simulink model "Snake_Robot_v2_wheels_test"  (R2022b)
settings: Solver=VariableStepAuto  StartTime=0.0  StopTime=300  RelTol=1e-5  AbsTol=1e-3  EnableMultiTasking=on
values from neighbouring files (symbols this model uses):
  amplitude = 2.5    [Snake_robot_parameters.m]
  frequency = 2    [Snake_robot_parameters.m]
  phase = 1.4    [Snake_robot_parameters.m]
undefined symbols (not defined in the file or in its folder): sigbuilder_block, X, Y, Z
libraries: sm_lib x134, nesl_utility x34, simulink x5, slpidlib x5, robotalgslib x1
(part 1 of 3)
settings Model: Creator=Antoine Masson  LastModifiedBy=Antoine Masson
settings SolverCC: AutoScaleAbsTol=off  MaxZcPerStep=1
settings DataIOCC: LimitDataPoints=on  MaxDataPoints=10000
settings OptimizationCC: LifeSpan=inf
settings DebuggingCC: UnconnectedInputMsg=warning  UnconnectedOutputMsg=warning  UnconnectedLineMsg=warning  AllowSymbolicDim=off  SFUnexpectedBacktrackingDiag=warning  SFNoUnconditionalDefaultTransitionDiag=warning  SFExecutionAtInitializationDiag=none  SFMachineParentedDataDiag=warning  ArithmeticOperatorsInVariantConditions=warning
settings ModelReferenceCC: EnableRefExpFcnMdlSchedulingChecks=on
settings SFSimCC: SimUseLocalCustomCode=off  CustomCodeUndefinedFunction=UseInterfaceOnly
settings RTWCC: RTWUseLocalCustomCode=off  DLArmComputeVersion=19.05
settings CodeAppCC: StateflowObjectComments=on
settings GRTTargetCC: TargetLangStandard=C89/C90 (ANSI)
settings ConfigComp: CovMetricSettings=dw  CovSaveCumulativeToWorkspaceVar=on  CovSaveSingleToWorkspaceVar=on  CovExternalEMLEnable=off  CovSFcnEnable=off
settings SimscapeCC: SimscapeLogType=all  SimscapeLogSimulationStatistics=on  SimscapeLogDataHistory=10000

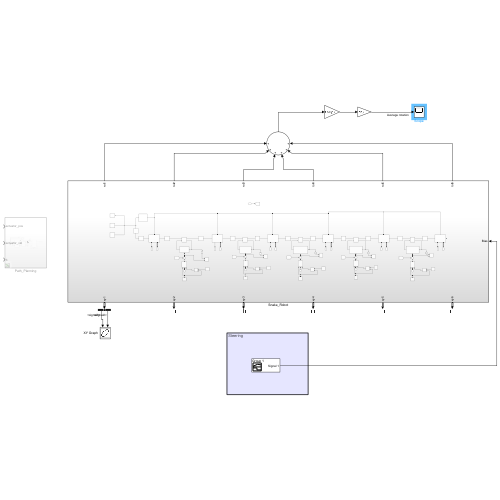
[thumbnail: Simulink's stored preview of the top-level diagram]
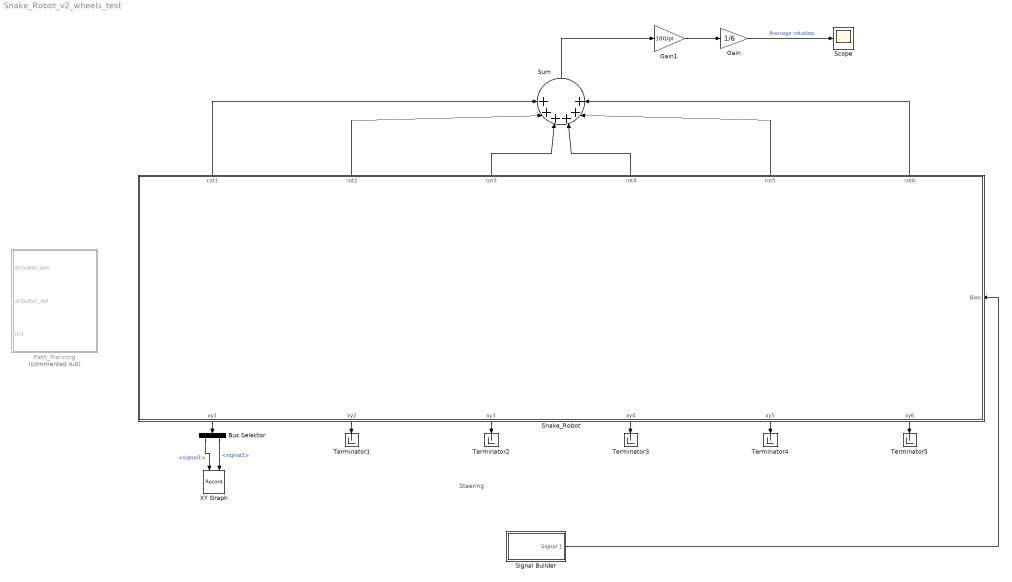
== system Snake_Robot_v2_wheels_test ==
  note: Steering
  Bus Selector : BusSelector  OutputSignals=signal1,signal2
  Gain : Gain  Gain=1/6
  Gain1 : Gain  Gain=180/pi
  Path_Planning : Subsystem  Commented=on
  Scope : Scope
  Signal Builder : Subsystem  Tag=STV Subsys  LoadFcn=sigbuilder_block('load');  StartFcn=sigbuilder_block('start');  StopFcn=sigbuilder_block('stop');  ClipboardFcn=sigbuilder_block('clipboard');  mask(Sigbuilder block){tuvar=[0:10]}
      mask help: Simulink:masks:SigbuilderBlock_MD
      mask init:
      | if ~strcmp(get_param(bdroot(gcbh),'SimulationStatus'),'stopped') tuvar = sigbuilder_block('maskInit'); end
      settings: CopyFcn=sigbuilder_block('copy');  DeleteFcn=sigbuilder_block('delete');  ModelCloseFcn=sigbuilder_block('modelClose');  PreSaveFcn=sigbuilder_block('preSave');  PauseFcn=sigbuilder_block('pause');  ContinueFcn=sigbuilder_block('continue');  NameChangeFcn=sigbuilder_block('namechange');  OpenFcn=sigbuilder_block('open',[407.4 143.4 550.8 400.2 ]);  CloseFcn=sigbuilder_block('close');
      mask Display: plot(0, 0, 100, 100,[2, 2, 32, 32, 2], [68, 8, 8, 68, 68],[32, 2], [38, 38], [32, 19, 2],[53, 60, 44], [32, 17, 17, 2],[16, 16, 31, 31]);txt = getActiveGroup(gcbh);text(2, 100, txt,'verticalAlignment', 'top');
  Snake_Robot : Subsystem
      settings: PortSchema="{\"entries\":[{\"content\":{\"sides\":[{\"content\":{\"connectorIds\":[]},\"type\":\"ConnectorPlacement.EquallySpacedRectSide\",\"uuid\":\"c8c3f42f-16ea-4b52-929c-6831ad7a0aa6\"},{\"content\":{\"connectorIds\":[\"In1\"],\"side\":\"RIGHT\"},\"type\":\"ConnectorPlacement.EquallySpacedRectSide\",\"uuid\":\"4df7dcd2-c9b7-4490-9994-4055ff239bfb\"},{\"content\":{\"connectorIds\":[\"Out7\",\"Out8\",\"Out9\",\"Out10\",\"Out11\",\"Out12\"],\"side\":\"TOP\"},\"type\":\"ConnectorPlacement.EquallySpacedRectSide\",\"uuid\":\"6c08f5c9-0650-48d0-8f84-c45eeca917d4\"},{\"content\":{\"connectorIds\":[\"Out1\",\"Out2\",\"Out3\",\"Out4\",\"Out5\",\"Out6\"],\"side\":\"BOTTOM\"},\"type\":\"ConnectorPlacement.EquallySpacedRectSide\",\"uuid\":\"57707fcd-8f3b-408f-aca2-991ac01d1cc1\"}]},\"type\":\"ConnectorPlacement.EquallySpacedConnector\",\"uuid\":\"e658f8a1-1b88-43a7-b7d0-c2a91e6742b3\"}],\"packageUris\":[\"http://schema.mathworks.com/mf0/Connector/R2020b\"],\"version\":\"1.0\"}"
  Sum : Sum  Inputs=++++++
  Terminator{1..5} (5 alike) : Terminator
  XY Graph : Record  FileSettingsInternal="{\"entries\":[{\"content\":{\"excelSettings\":{\"content\":{},\"type\":\"Streamout.ExcelSettings\"}},\"type\":\"Streamout.FileSettingStorage\",\"uuid\":\"84e75361-550c-4476-9ed0-9b3ec4275fe3\"}],\"packageUris\":[\"http://schema.mathworks.com/mf0/streamout_blocks/R2020a\"],\"version\":\"1.0\"}"  Layout=[1 1]  SignalsInternal="{\"entries\":[{\"content\":{\"signals\":[{\"content\":{\"blockPath\":[\"Snake_Robot_v2_wheels_test/XY Graph\"],\"channel\":[],\"dimensions\":[1,1],\"domain\":\"Snake_Robot_v2_wheels_test/XY Graph\",\"lineColor\":\"#a2142f\",\"plots\":[1],\"port\":1,\"sid\":[\"\"],\"signalID\":51,\"signalName\":\"<signal1>\"},\"type\":\"RecordBlkView.Signal\",\"uuid\":\"4d76fd36-35a8-4129-8bfe-1a376abbe28c\"},{\"content\":{\"blockPath\":[\"Snake_Robot_v2_wheels_test/XY Graph\"],\"channel\":[],\"dimensions\":[1,1],\"domain\":\"Snake_Robot_v2_wheels_test/XY Graph\",\"lineColor\":\"#139fff\",\"plots\":[1],\"port\":2,\"sid\":[\"\"],\"signalID\":56,\"signalName\":\"<signal2>\"},\"type\":\"RecordBlkView.Signal\",\"uuid\":\"5b063d72-9b00-41f5-95b4-b99475b325a9\"}]},\"type\":\"RecordBlkView.InputSignals\",\"uuid\":\"10acdae6-4853-4f6f-9407-9f8053fa8a6d\"}],\"packageUris\":[\"http://schema.mathworks.com/mf0/streamout_blocks/R2020a\"],\"version\":\"1.0\"}"  VisualizationBindings="{\"xyplotplugin\":{\"info\":[{\"series\":[{\"bindingParametersList\":[{\"parameter\":\"X-Axis\",\"signalID\":51,\"signalName\":\"<signal1>\"},{\"parameter\":\"Y-Axis\",\"signalID\":56,\"signalName\":\"<signal2>\"}],\"seriesID\":31576}],\"subplotID\":1}]}}"  CompatibilityTag=XY
  wires:
  Signal Builder/1(Signal 1) -> Snake_Robot/1(Bias)
  Sum/1 -> Gain1/1
  Snake_Robot/7(rot1) -> Sum/1
  Snake_Robot/8(rot2) -> Sum/2
  Snake_Robot/9(rot3) -> Sum/3
  Snake_Robot/10(rot4) -> Sum/4
  Snake_Robot/11(rot5) -> Sum/5
  Snake_Robot/12(rot6) -> Sum/6
  Snake_Robot/1(xy1) -> Bus Selector/1
  Snake_Robot/2(xy2) -> Terminator1/1
  Snake_Robot/3(xy3) -> Terminator2/1
  Snake_Robot/4(xy4) -> Terminator3/1
  Snake_Robot/5(xy5) -> Terminator4/1
  Snake_Robot/6(xy6) -> Terminator5/1
  Gain/1 -> Scope/1  "Average rotation"
  Gain1/1 -> Gain/1
  Bus Selector/1 -> XY Graph/1  "<signal1>"
  Bus Selector/2 -> XY Graph/2  "<signal2>"

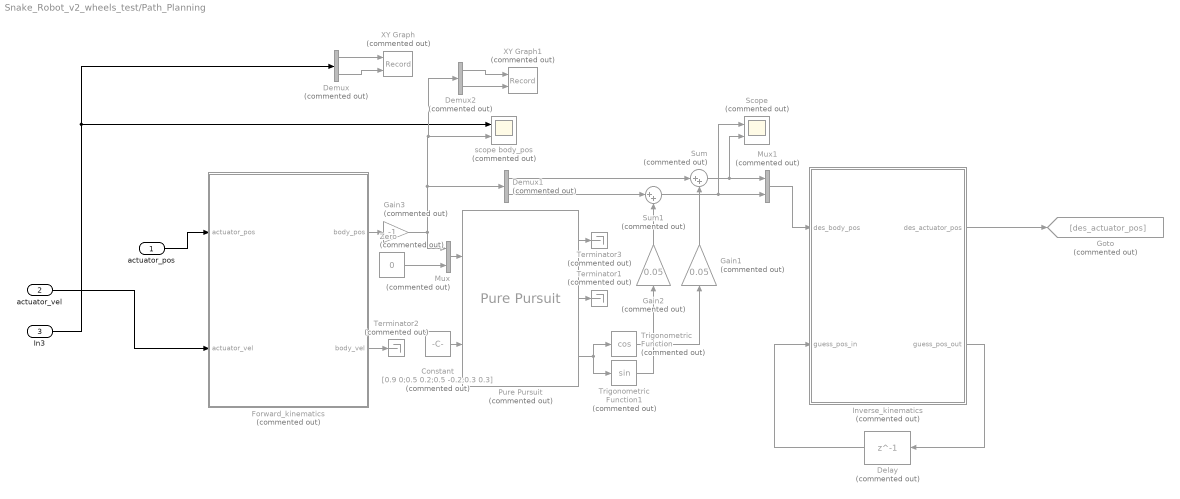
== system Snake_Robot_v2_wheels_test/Path_Planning ==
  actuator_pos : Inport
  actuator_vel : Inport  Port=2
  In3 : Inport  Port=3
  Constant : Constant  Commented=on  Value=[0.9 0;0.5 0.2;0.5 -0.2;0.3 0.3]
  Delay : Delay  Commented=on  DelayLength=1  InitialCondition=zeros(3,1)  SampleTime=0.01
  Demux : Demux  Commented=on  Outputs=2
  Demux1 : Demux  Commented=on  Outputs=2
  Demux2 : Demux  Commented=on  Outputs=2
  Forward_kinematics : MATLAB Function  Commented=on  TreatAsAtomicUnit=on
  Gain1 : Gain  Commented=on  Gain=0.05
  Gain2 : Gain  Commented=on  Gain=0.05
  Gain3 : Gain  Commented=on  Gain=-1
  Goto : Goto  Commented=on  GotoTag=des_actuator_pos
  Inverse_kinematics : MATLAB Function  Commented=on  TreatAsAtomicUnit=on
  Mux : Mux  Commented=on  Inputs=2
  Mux1 : Mux  Commented=on  Inputs=2
  Pure Pursuit : robotalgslib/Pure Pursuit  Commented=on  DesiredLinearVelocity=0.05  MaxAngularVelocity=1  LookaheadDistance=0.05  TargetDirPort=on  SimulateUsing=Code generation
      settings: LibrarySourceBlock=navlib/Control Algorithms/Pure Pursuit
  Scope : Scope  Commented=on  NumInputPorts=2
  Sum : Sum  Commented=on  Inputs=|++
  Sum1 : Sum  Commented=on  Inputs=|++
  Terminator1 : Terminator  Commented=on
  Terminator2 : Terminator  Commented=on
  Terminator3 : Terminator  Commented=on
  Trigonometric Function : Trigonometry  Commented=on  Operator=cos
  Trigonometric Function1 : Trigonometry  Commented=on
  XY Graph : Record  Commented=on  FileSettingsInternal="{\"entries\":[{\"content\":{\"excelSettings\":{\"content\":{},\"type\":\"Streamout.ExcelSettings\"}},\"type\":\"Streamout.FileSettingStorage\",\"uuid\":\"73da843e-60dd-4a33-b665-f9131d8271e1\"}],\"packageUris\":[\"http://schema.mathworks.com/mf0/streamout_blocks/R2020a\"],\"version\":\"1.0\"}"  Layout=[1 1]  SignalsInternal="{\"entries\":[{\"content\":{\"signals\":[{\"content\":{\"blockPath\":[\"Snake_Robot_v2_wheels_test/Path_Planning/XY Graph\"],\"channel\":[],\"dimensions\":[1],\"domain\":\"Snake_Robot_v2_wheels_test/Path_Planning/XY Graph\",\"lineColor\":\"#a2142f\",\"plots\":[1],\"port\":1,\"sid\":[],\"signalID\":16,\"signalName\":\"Demux:1\"},\"type\":\"RecordBlkView.Signal\",\"uuid\":\"8e68c205-c0fd-447d-ace0-da6efb5c1fbf\"},{\"content\":{\"blockPath\":[\"Snake_Robot_v2_wheels_test/Path_Planning/XY Graph\"],\"channel\":[],\"dimensions\":[1],\"domain\":\"Snake_Robot_v2_wheels_test/Path_Planning/XY Graph\",\"lineColor\":\"#139fff\",\"plots\":[1],\"port\":2,\"sid\":[],\"signalID\":19,\"signalName\":\"Demux:2\"},\"type\":\"RecordBlkView.Signal\",\"uuid\":\"8eb45edb-93bd-48a6-8f31-f79372ca3dc9\"}]},\"type\":\"RecordBlkView.InputSignals\",\"uuid\":\"d43a9e34-8350-459e-ae19-866886e7c1fb\"}],\"packageUris\":[\"http://schema.mathworks.com/mf0/streamout_blocks/R2020a\"],\"version\":\"1.0\"}"  VisualizationBindings="{\"xyplotplugin\":{\"info\":[{\"series\":[{\"bindingParametersList\":[{\"parameter\":\"X-Axis\",\"signalID\":16,\"signalName\":\"Demux:1\"},{\"parameter\":\"Y-Axis\",\"signalID\":19,\"signalName\":\"Demux:2\"}],\"seriesID\":12260}],\"subplotID\":1}]}}"  CompatibilityTag=XY
  XY Graph1 : Record  Commented=on  FileSettingsInternal="{\"entries\":[{\"content\":{\"excelSettings\":{\"content\":{},\"type\":\"Streamout.ExcelSettings\"}},\"type\":\"Streamout.FileSettingStorage\",\"uuid\":\"52cbc1bb-b168-4d3a-81e4-39640940caf6\"}],\"packageUris\":[\"http://schema.mathworks.com/mf0/streamout_blocks/R2020a\"],\"version\":\"1.0\"}"  Layout=[1 1]  SignalsInternal="{\"entries\":[{\"content\":{\"signals\":[{\"content\":{\"blockPath\":[\"Snake_Robot_v2_wheels_test/Path_Planning/XY Graph1\"],\"channel\":[],\"dimensions\":[1,1],\"domain\":\"Snake_Robot_v2_wheels_test/Path_Planning/XY Graph1\",\"lineColor\":\"#a2142f\",\"plots\":[1],\"port\":1,\"sid\":[],\"signalID\":8,\"signalName\":\"Demux2:1\"},\"type\":\"RecordBlkView.Signal\",\"uuid\":\"6807b1ac-bdd6-4ace-a695-6e3cb940d5f2\"},{\"content\":{\"blockPath\":[\"Snake_Robot_v2_wheels_test/Path_Planning/XY Graph1\"],\"channel\":[],\"dimensions\":[1,1],\"domain\":\"Snake_Robot_v2_wheels_test/Path_Planning/XY Graph1\",\"lineColor\":\"#139fff\",\"plots\":[1],\"port\":2,\"sid\":[],\"signalID\":11,\"signalName\":\"Demux2:2\"},\"type\":\"RecordBlkView.Signal\",\"uuid\":\"ed18573f-74af-480a-a61e-83f3faac892a\"}]},\"type\":\"RecordBlkView.InputSignals\",\"uuid\":\"ad915e20-bbb1-4588-94b6-02e62a7d6124\"}],\"packageUris\":[\"http://schema.mathworks.com/mf0/streamout_blocks/R2020a\"],\"version\":\"1.0\"}"  VisualizationBindings="{\"xyplotplugin\":{\"info\":[{\"series\":[{\"bindingParametersList\":[{\"parameter\":\"X-Axis\",\"signalID\":8,\"signalName\":\"Demux2:1\"},{\"parameter\":\"Y-Axis\",\"signalID\":11,\"signalName\":\"Demux2:2\"}],\"seriesID\":53918}],\"subplotID\":1}]}}"  CompatibilityTag=XY
  Zero : Constant  Commented=on  Value=0  OutDataTypeStr=Inherit: Inherit via back propagation
  scope body_pos : Scope  Commented=on  NumInputPorts=2
  wires:
  Forward_kinematics/1(body_pos) -> Gain3/1
  Trigonometric Function/1 -> Gain1/1
  Demux1/2 -> Sum1/1
  Sum/1 -> Scope/2, Mux1/1
  Inverse_kinematics/1(des_actuator_pos) -> Goto/1
  Constant/1 -> Pure Pursuit/2
  Pure Pursuit/3 -> Trigonometric Function/1, Trigonometric Function1/1
  Mux/1 -> Pure Pursuit/1
  In3/1 -> Demux/1, scope body_pos/1
  Mux1/1 -> Inverse_kinematics/1(des_body_pos)
  Forward_kinematics/2(body_vel) -> Terminator2/1
  Demux2/1 -> XY Graph1/1
  Sum1/1 -> Scope/1, Mux1/2
  Gain2/1 -> Sum1/2
  Gain1/1 -> Sum/2
  Trigonometric Function1/1 -> Gain2/1
  Delay/1 -> Inverse_kinematics/2(guess_pos_in)
  actuator_vel/1 -> Forward_kinematics/2(actuator_vel)
  Inverse_kinematics/2(guess_pos_out) -> Delay/1
  Gain3/1 -> Mux/1, Demux2/1, scope body_pos/2, Demux1/1
  Demux1/1 -> Sum/1
  Zero/1 -> Mux/2
  Pure Pursuit/2 -> Terminator1/1
  Demux2/2 -> XY Graph1/2
  Pure Pursuit/1 -> Terminator3/1
  Demux/1 -> XY Graph/1
  Demux/2 -> XY Graph/2
  actuator_pos/1 -> Forward_kinematics/1(actuator_pos)

== system Snake_Robot_v2_wheels_test/Signal Builder ==
  Demux : Demux  Tag=STV Demux  Outputs=1
      settings: DisplayOption=none
  FromWs : FromWorkspace  Tag=STV FromWs  VariableName=tuvar
      SigBuilderData=|
      | common.afterFinalStr = 'Extrapolate'
      | common.sampleTime = 0
      | dataSet.timeRange = [0 60]
      | dataSet.name = 'Group 1'
      | sbobj.Groups.Name = 'Group 1'
      | sbobj.Groups.Signals.Name = 'Signal 1'
      | sbobj.Groups.Signals.XData = [0 15 19 23 35 40 45 60]
      | sbobj.Groups.Signals.YData = [0 0 -0.3 0 0 0.3 0 0]
      | sbobj.Groups.TimeRange = [0 60]
  Signal 1 : Outport  Tag=STV Outport
  wires:
  Demux/1 -> Signal 1/1
  FromWs/1 -> Demux/1

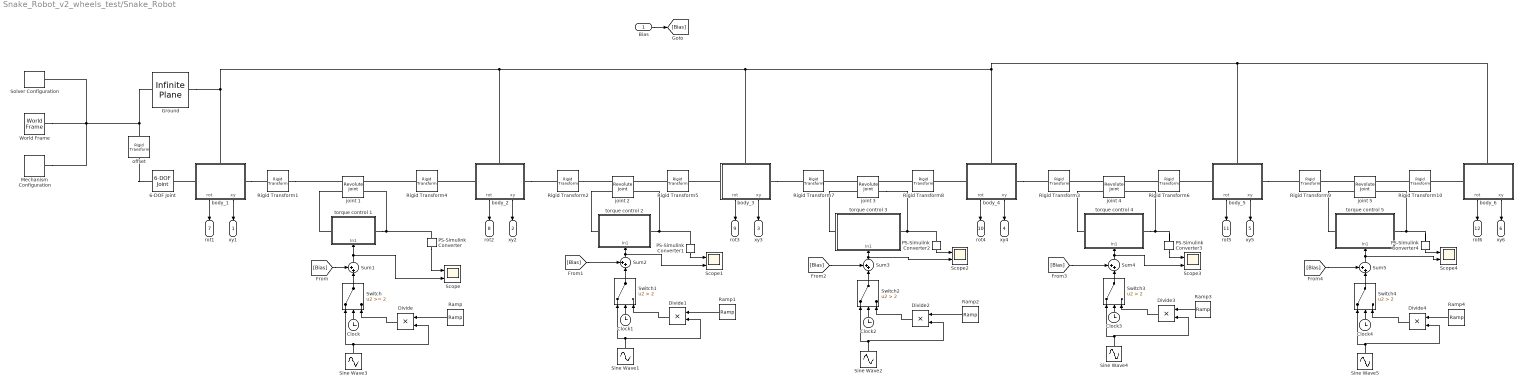
== system Snake_Robot_v2_wheels_test/Snake_Robot ==
  Bias : Inport
  6-DOF Joint : sm_lib/Joints/6-DOF Joint  JointMode=Normal  SenseConstraintForce=off  SenseConstraintForceX=off  SenseConstraintForceY=off  SenseConstraintForceZ=off  SenseConstraintTorque=off  SenseConstraintTorqueX=off  SenseConstraintTorqueY=off  SenseConstraintTorqueZ=off  SenseTotalForce=off  SenseTotalForceX=off  SenseTotalForceY=off  SenseTotalForceZ=off  SenseTotalTorque=off  SenseTotalTorqueX=off  SenseTotalTorqueY=off  SenseTotalTorqueZ=off  CompositeWrenchDir=FollowerOnBase  CompositeWrenchFrame=BaseFrame  PxEquilibriumPosition=0  PxEquilibriumPositionUnits=m  PxSpringStiffness=0  PxSpringStiffnessUnits=N/m  PxDampingCoefficient=0  PxDampingCoefficientUnits=N/(m/s)  PxTorqueActuationMode=NoTorque  PxMotionActuationMode=ComputedMotion  PxSensePosition=off  PxSenseVelocity=off  PxSenseAcceleration=off  PxSenseTorqueForce=off  PxSenseLowerLimitTorqueForce=off  PxSenseUpperLimitTorqueForce=off  PxLowerLimitSpecify=off  PxLowerLimitBound=-1  PxLowerLimitBoundUnits=m  PxLowerLimitStiffness=1e6  PxLowerLimitStiffnessUnits=N/m  PxLowerLimitDamping=1e3  PxLowerLimitDampingUnits=N/(m/s)  PxLowerLimitTransitionRegionWidth=1e-4  PxLowerLimitTransitionRegionWidthUnits=m  PxUpperLimitSpecify=off  PxUpperLimitBound=1  PxUpperLimitBoundUnits=m  PxUpperLimitStiffness=1e6  PxUpperLimitStiffnessUnits=N/m  PxUpperLimitDamping=1e3  PxUpperLimitDampingUnits=N/(m/s)  PxUpperLimitTransitionRegionWidth=1e-4  PxUpperLimitTransitionRegionWidthUnits=m  PxPositionTargetSpecify=off  PxPositionTargetPriority=High  PxPositionTargetValue=0  PxPositionTargetValueUnits=m  PxVelocityTargetSpecify=off  PxVelocityTargetPriority=High  PxVelocityTargetValue=0  PxVelocityTargetValueUnits=m/s  PyEquilibriumPosition=0  PyEquilibriumPositionUnits=m  PySpringStiffness=0  PySpringStiffnessUnits=N/m  PyDampingCoefficient=0  PyDampingCoefficientUnits=N/(m/s)  PyTorqueActuationMode=NoTorque  PyMotionActuationMode=ComputedMotion  PySensePosition=off  PySenseVelocity=off  PySenseAcceleration=off  PySenseTorqueForce=off  PySenseLowerLimitTorqueForce=off  PySenseUpperLimitTorqueForce=off  PyLowerLimitSpecify=off  PyLowerLimitBound=-1  PyLowerLimitBoundUnits=m  PyLowerLimitStiffness=1e6  PyLowerLimitStiffnessUnits=N/m  PyLowerLimitDamping=1e3  PyLowerLimitDampingUnits=N/(m/s)  PyLowerLimitTransitionRegionWidth=1e-4  PyLowerLimitTransitionRegionWidthUnits=m  PyUpperLimitSpecify=off  PyUpperLimitBound=1  PyUpperLimitBoundUnits=m  PyUpperLimitStiffness=1e6  PyUpperLimitStiffnessUnits=N/m  PyUpperLimitDamping=1e3  PyUpperLimitDampingUnits=N/(m/s)  PyUpperLimitTransitionRegionWidth=1e-4  PyUpperLimitTransitionRegionWidthUnits=m  PyPositionTargetSpecify=off  PyPositionTargetPriority=High  PyPositionTargetValue=0  PyPositionTargetValueUnits=m  PyVelocityTargetSpecify=off  PyVelocityTargetPriority=High  PyVelocityTargetValue=0  PyVelocityTargetValueUnits=m/s  PzEquilibriumPosition=0  PzEquilibriumPositionUnits=m  PzSpringStiffness=0  PzSpringStiffnessUnits=N/m  PzDampingCoefficient=0  PzDampingCoefficientUnits=N/(m/s)  PzTorqueActuationMode=NoTorque  PzMotionActuationMode=ComputedMotion  PzSensePosition=off  PzSenseVelocity=off  PzSenseAcceleration=off  PzSenseTorqueForce=off  PzSenseLowerLimitTorqueForce=off  PzSenseUpperLimitTorqueForce=off  PzLowerLimitSpecify=off  PzLowerLimitBound=-1  PzLowerLimitBoundUnits=m  PzLowerLimitStiffness=1e6  PzLowerLimitStiffnessUnits=N/m  PzLowerLimitDamping=1e3  PzLowerLimitDampingUnits=N/(m/s)  PzLowerLimitTransitionRegionWidth=1e-4  PzLowerLimitTransitionRegionWidthUnits=m  PzUpperLimitSpecify=off  PzUpperLimitBound=1  PzUpperLimitBoundUnits=m  PzUpperLimitStiffness=1e6  PzUpperLimitStiffnessUnits=N/m  PzUpperLimitDamping=1e3  PzUpperLimitDampingUnits=N/(m/s)  PzUpperLimitTransitionRegionWidth=1e-4  PzUpperLimitTransitionRegionWidthUnits=m  PzPositionTargetSpecify=off  PzPositionTargetPriority=High  PzPositionTargetValue=0  PzPositionTargetValueUnits=m  PzVelocityTargetSpecify=off  PzVelocityTargetPriority=High  PzVelocityTargetValue=0  PzVelocityTargetValueUnits=m/s  SphEqPosRotationMethod=None  SphEqPosRotationAngleUnits=deg  SphEqPosRotationStandardAxis=+Z  SphEqPosRotationAngle=0.0  SphEqPosRotationArbitraryAxis=[0 0 1]  SphEqPosFollAlignAxisA=+X  SphEqPosBaseAlignAxisA=+Y  SphEqPosFollAlignAxisB=+Y  SphEqPosBaseAlignAxisB=+Z  SphEqPosRotationSequenceAxes=FollowerAxes  SphEqPosRotationSequence=XYX  SphEqPosRotationSequenceAngles=[0 0 0]  SphEqPosRotationSequenceAnglesUnits=deg  SphEqPosRotationMatrix=[1 0 0; 0 1 0; 0 0 1]  SphEqPosQuaternion=[1 0 0 0]  SphSpringStiffness=0  SphSpringStiffnessUnits=N*m/deg  SphDampingCoefficient=0  SphDampingCoefficientUnits=N*m/(deg/s)  SphActuateTorqueX=off  SphActuateTorqueY=off  SphActuateTorqueZ=off  SphActuateTorque=off  SphTorqueActuationMode=NoTorque  SphMotionActuationMode=ComputedMotion  SphActuationFrame=BaseFrame  SphSensePosition=off  SphSenseVelocityX=off  SphSenseVelocityY=off  SphSenseVelocityZ=off  SphSenseVelocity=off  SphSenseAccelerationX=off  SphSenseAccelerationY=off  SphSenseAccelerationZ=off  SphSenseAcceleration=off  SphSenseTorqueX=off  SphSenseTorqueY=off  SphSenseTorqueZ=off  SphSenseTorqueForce=off  SphSenseLowerLimitTorqueMag=off  SphSenseUpperLimitTorqueMag=off  SphSensingFrame=BaseFrame  SphLowerLimitSpecify=off  SphLowerLimitBound=15  SphLowerLimitBoundUnits=deg  SphLowerLimitStiffness=1e4  SphLowerLimitStiffnessUnits=N*m/deg  SphLowerLimitDamping=10  SphLowerLimitDampingUnits=N*m/(deg/s)  SphLowerLimitTransitionRegionWidth=0.1  SphLowerLimitTransitionRegionWidthUnits=deg  SphUpperLimitSpecify=off  SphUpperLimitBound=45  SphUpperLimitBoundUnits=deg  SphUpperLimitStiffness=1e4  SphUpperLimitStiffnessUnits=N*m/deg  SphUpperLimitDamping=10  SphUpperLimitDampingUnits=N*m/(deg/s)  SphUpperLimitTransitionRegionWidth=0.1  SphUpperLimitTransitionRegionWidthUnits=deg  SphPositionTargetRotationMethod=None  SphPositionTargetRotationAngleUnits=deg  SphPositionTargetRotationStandardAxis=+Z  SphPositionTargetRotationAngle=0.0  SphPositionTargetRotationArbitraryAxis=[0 0 1]  SphPositionTargetFollAlignAxisA=+X  SphPositionTargetBaseAlignAxisA=+Y  SphPositionTargetFollAlignAxisB=+Y  SphPositionTargetBaseAlignAxisB=+Z  SphPositionTargetRotationSequenceAxes=FollowerAxes  SphPositionTargetRotationSequence=XYX  SphPositionTargetRotationSequenceAngles=[0 0 0]  SphPositionTargetRotationSequenceAnglesUnits=deg  SphPositionTargetRotationMatrix=[1 0 0; 0 1 0; 0 0 1]  SphPositionTargetQuaternion=[1 0 0 0]  SphPositionTargetSpecify=off  SphPositionTargetPriority=High  SphVelocityTargetValue=[0 0 0]  SphVelocityTargetValueUnits=deg/s  SphVelocityTargetSpecify=off  SphVelocityTargetPriority=High  SphVelocityTargetInFollowerFrame=on
  Clock{,1..4} (5 alike) : Clock
  Divide{,1..4} (5 alike) : Product  Inputs=**
  Ground : sm_lib/Curves and Surfaces/Infinite Plane  GraphicType=Rectangle  GraphicPlaneWidth=20  GraphicPlaneWidthUnits=m  GraphicPlaneHeight=20  GraphicPlaneHeightUnits=m  GraphicVisPropType=SimpleVisualProperties  GraphicDiffuseColor=[1 1 1]  GraphicOpacity=1  GraphicSpecularColor=[0.5 0.5 0.5 1.0]  GraphicAmbientColor=[0.15 0.15 0.15 1.0]  GraphicEmissiveColor=[0.0 0.0 0.0 1.0]  GraphicShininess=75
  Mechanism Configuration : sm_lib/Utilities/Mechanism Configuration  UniformGravity=Constant  GravityVector=[0 0 -9.80665]  GravityUnits=m/s^2  LinearizationDelta=0.001  JointModeTransitionNonlinearIterations=2
  PS-Simulink Converter{,1..4} (5 alike) : nesl_utility/PS-Simulink Converter  PhysicalDomain=network_engine_domain  SubClassName=ps_output  LeftPortType=input  RightPortType=output  PseudoPeriodic=off  Frequencies=[]  VectorFormat=inherit  Unit=inherit  AffineConversion=off
  Ramp{,1..4} (5 alike) : simulink/Sources/Ramp  slope=0.5  start=0  InitialOutput=0
  Rigid Transform{1..10} (10 alike) : sm_lib/Frames and Transforms/Rigid Transform  TranslationMethod=Cartesian  TranslationStandardOffset=0  TranslationLengthUnit=m  TranslationStandardAxis=+Z  TranslationCartesianOffset=[0.05 0 0]  TranslationROffset=0  TranslationROffsetUnits=m  TranslationZOffset=0  TranslationZOffsetUnits=m  TranslationThetaOffset=0  TranslationThetaOffsetUnits=deg  RotationMethod=None  RotationAngleUnits=deg  RotationStandardAxis=+Z  RotationAngle=0.0  RotationArbitraryAxis=[0 0 1]  FollAlignAxisA=+X  BaseAlignAxisA=+Y  FollAlignAxisB=+Y  BaseAlignAxisB=+Z  RotationSequenceAxes=FollowerAxes  RotationSequence=XYX  RotationSequenceAngles=[0 0 0]  RotationSequenceAnglesUnits=deg  RotationMatrix=[1 0 0; 0 1 0; 0 0 1]  Quaternion=[1 0 0 0]
  Scope{,1..4} (5 alike) : Scope  NumInputPorts=2
  Sine Wave1 : Sin  Amplitude=amplitude  Frequency=frequency  Phase=1*phase  SampleTime=0.01
  Sine Wave2 : Sin  Amplitude=amplitude  Frequency=frequency  Phase=2*phase  SampleTime=0.01
  Sine Wave3 : Sin  Amplitude=amplitude  Frequency=frequency  Phase=0*phase  SampleTime=0.01
  Sine Wave4 : Sin  Amplitude=amplitude  Frequency=frequency  Phase=3*phase  SampleTime=0.01
  Sine Wave5 : Sin  Amplitude=amplitude  Frequency=frequency  Phase=4*phase  SampleTime=0.01
  Solver Configuration : nesl_utility/Solver Configuration  PhysicalDomain=network_engine_domain  SubClassName=solver  LeftPortType=input  RightPortType=generic  Tones=[]  Harmonics=[]  SimulateNoise=off  Profile=off  UseLocalSampling=off  EnableSwitchedLinearOptims=on  FrequencyDomain=off  UseCCode=off  RelTol=0.001  AbsTol=1e-06  MinStep=1e-09  ToWorkspace=off  RevertToSquareIcSolve=off  NumHomotopyIterations=100  PhasorMode=off  PhasorModeNumHarmonics=1  ConsistencySolver=NEWTON_XTOL_AFTER_FTOL  IndexReductionMethod=DerivativeReplacement  DoDC=off  ResidualTolerance=1e-09  ConsistencyTolSource=GLOBAL  ConsistencyAbsTol=0.001  ConsistencyRelTol=0.001  ConsistencyTolFactor=0.001  UseLocalSolver=off  LocalSolverChoice=NE_BACKWARD_EULER_ADVANCER  ResolveIndetEquations=on  FunctionEvalNumThread=1  LocalSolverSampleTime=0.001  DoFixedCost=off  MaxNonlinIter=3  MaxModeIter=2  ComputeImpulses=off  ImpulseIterations=2  LinearAlgebra=Sparse  LinearAlgebraNumThread=0  EquationFormulation=NE_TIME_EF  DelaysMemoryBudget=1024  AutomaticFiltering=on  FilteringTimeConstant=0.001  PartitionStorageMethod=AS_NEEDED  PartitionMemoryBudget=1024  PartitionMethod=FAST
  Sum{1..5} (5 alike) : Sum  Inputs=++|
  Switch : Switch  Threshold=2  SaturateOnIntegerOverflow=off  InputSameDT=off
  Switch{1..4} (4 alike) : Switch  Criteria=u2 > Threshold  Threshold=2  SaturateOnIntegerOverflow=off  InputSameDT=off
  World Frame : sm_lib/Frames and Transforms/World Frame
  body_1 : Subsystem
      settings: PortSchema="{\"entries\":[{\"content\":{\"sides\":[{\"content\":{\"connectorIds\":[\"LConn1\"]},\"type\":\"ConnectorPlacement.EquallySpacedRectSide\",\"uuid\":\"751caf70-fea4-4832-96d1-cfb89594f882\"},{\"content\":{\"connectorIds\":[\"RConn1\"],\"side\":\"RIGHT\"},\"type\":\"ConnectorPlacement.EquallySpacedRectSide\",\"uuid\":\"f4256cb0-7155-4962-9e91-24184222dcac\"},{\"content\":{\"connectorIds\":[\"LConn2\"],\"side\":\"TOP\"},\"type\":\"ConnectorPlacement.EquallySpacedRectSide\",\"uuid\":\"795803ba-ad55-452c-8522-189aeb3dc475\"},{\"content\":{\"connectorIds\":[\"Out1\",\"Out2\"],\"side\":\"BOTTOM\"},\"type\":\"ConnectorPlacement.EquallySpacedRectSide\",\"uuid\":\"40385723-46d7-44c7-bad8-75426342e5d4\"}]},\"type\":\"ConnectorPlacement.EquallySpacedConnector\",\"uuid\":\"3814bf41-4d16-483c-99d1-47665b43720b\"}],\"packageUris\":[\"http://schema.mathworks.com/mf0/Connector/R2020b\"],\"version\":\"1.0\"}"
  body_2 : Subsystem
      settings: PortSchema="{\"entries\":[{\"content\":{\"sides\":[{\"content\":{\"connectorIds\":[\"LConn1\"]},\"type\":\"ConnectorPlacement.EquallySpacedRectSide\",\"uuid\":\"751caf70-fea4-4832-96d1-cfb89594f882\"},{\"content\":{\"connectorIds\":[\"RConn1\"],\"side\":\"RIGHT\"},\"type\":\"ConnectorPlacement.EquallySpacedRectSide\",\"uuid\":\"f4256cb0-7155-4962-9e91-24184222dcac\"},{\"content\":{\"connectorIds\":[\"LConn2\"],\"side\":\"TOP\"},\"type\":\"ConnectorPlacement.EquallySpacedRectSide\",\"uuid\":\"795803ba-ad55-452c-8522-189aeb3dc475\"},{\"content\":{\"connectorIds\":[\"Out1\",\"Out2\"],\"side\":\"BOTTOM\"},\"type\":\"ConnectorPlacement.EquallySpacedRectSide\",\"uuid\":\"40385723-46d7-44c7-bad8-75426342e5d4\"}]},\"type\":\"ConnectorPlacement.EquallySpacedConnector\",\"uuid\":\"3814bf41-4d16-483c-99d1-47665b43720b\"}],\"packageUris\":[\"http://schema.mathworks.com/mf0/Connector/R2020b\"],\"version\":\"1.0\"}"
  body_3 : Subsystem
      settings: PortSchema="{\"entries\":[{\"content\":{\"sides\":[{\"content\":{\"connectorIds\":[\"LConn1\"]},\"type\":\"ConnectorPlacement.EquallySpacedRectSide\",\"uuid\":\"751caf70-fea4-4832-96d1-cfb89594f882\"},{\"content\":{\"connectorIds\":[\"RConn1\"],\"side\":\"RIGHT\"},\"type\":\"ConnectorPlacement.EquallySpacedRectSide\",\"uuid\":\"f4256cb0-7155-4962-9e91-24184222dcac\"},{\"content\":{\"connectorIds\":[\"LConn2\"],\"side\":\"TOP\"},\"type\":\"ConnectorPlacement.EquallySpacedRectSide\",\"uuid\":\"795803ba-ad55-452c-8522-189aeb3dc475\"},{\"content\":{\"connectorIds\":[\"Out1\",\"Out2\"],\"side\":\"BOTTOM\"},\"type\":\"ConnectorPlacement.EquallySpacedRectSide\",\"uuid\":\"40385723-46d7-44c7-bad8-75426342e5d4\"}]},\"type\":\"ConnectorPlacement.EquallySpacedConnector\",\"uuid\":\"3814bf41-4d16-483c-99d1-47665b43720b\"}],\"packageUris\":[\"http://schema.mathworks.com/mf0/Connector/R2020b\"],\"version\":\"1.0\"}"
  body_4 : Subsystem
      settings: PortSchema="{\"entries\":[{\"content\":{\"sides\":[{\"content\":{\"connectorIds\":[\"LConn1\"]},\"type\":\"ConnectorPlacement.EquallySpacedRectSide\",\"uuid\":\"751caf70-fea4-4832-96d1-cfb89594f882\"},{\"content\":{\"connectorIds\":[\"RConn1\"],\"side\":\"RIGHT\"},\"type\":\"ConnectorPlacement.EquallySpacedRectSide\",\"uuid\":\"f4256cb0-7155-4962-9e91-24184222dcac\"},{\"content\":{\"connectorIds\":[\"LConn2\"],\"side\":\"TOP\"},\"type\":\"ConnectorPlacement.EquallySpacedRectSide\",\"uuid\":\"795803ba-ad55-452c-8522-189aeb3dc475\"},{\"content\":{\"connectorIds\":[\"Out1\",\"Out2\"],\"side\":\"BOTTOM\"},\"type\":\"ConnectorPlacement.EquallySpacedRectSide\",\"uuid\":\"40385723-46d7-44c7-bad8-75426342e5d4\"}]},\"type\":\"ConnectorPlacement.EquallySpacedConnector\",\"uuid\":\"3814bf41-4d16-483c-99d1-47665b43720b\"}],\"packageUris\":[\"http://schema.mathworks.com/mf0/Connector/R2020b\"],\"version\":\"1.0\"}"
  body_5 : Subsystem
      settings: PortSchema="{\"entries\":[{\"content\":{\"sides\":[{\"content\":{\"connectorIds\":[\"LConn1\"]},\"type\":\"ConnectorPlacement.EquallySpacedRectSide\",\"uuid\":\"751caf70-fea4-4832-96d1-cfb89594f882\"},{\"content\":{\"connectorIds\":[\"RConn1\"],\"side\":\"RIGHT\"},\"type\":\"ConnectorPlacement.EquallySpacedRectSide\",\"uuid\":\"f4256cb0-7155-4962-9e91-24184222dcac\"},{\"content\":{\"connectorIds\":[\"LConn2\"],\"side\":\"TOP\"},\"type\":\"ConnectorPlacement.EquallySpacedRectSide\",\"uuid\":\"795803ba-ad55-452c-8522-189aeb3dc475\"},{\"content\":{\"connectorIds\":[\"Out1\",\"Out2\"],\"side\":\"BOTTOM\"},\"type\":\"ConnectorPlacement.EquallySpacedRectSide\",\"uuid\":\"40385723-46d7-44c7-bad8-75426342e5d4\"}]},\"type\":\"ConnectorPlacement.EquallySpacedConnector\",\"uuid\":\"3814bf41-4d16-483c-99d1-47665b43720b\"}],\"packageUris\":[\"http://schema.mathworks.com/mf0/Connector/R2020b\"],\"version\":\"1.0\"}"
  body_6 : Subsystem
      settings: PortSchema="{\"entries\":[{\"content\":{\"sides\":[{\"content\":{\"connectorIds\":[\"LConn1\"]},\"type\":\"ConnectorPlacement.EquallySpacedRectSide\",\"uuid\":\"751caf70-fea4-4832-96d1-cfb89594f882\"},{\"content\":{\"connectorIds\":[\"RConn1\"],\"side\":\"RIGHT\"},\"type\":\"ConnectorPlacement.EquallySpacedRectSide\",\"uuid\":\"f4256cb0-7155-4962-9e91-24184222dcac\"},{\"content\":{\"connectorIds\":[\"LConn2\"],\"side\":\"TOP\"},\"type\":\"ConnectorPlacement.EquallySpacedRectSide\",\"uuid\":\"795803ba-ad55-452c-8522-189aeb3dc475\"},{\"content\":{\"connectorIds\":[\"Out1\",\"Out2\"],\"side\":\"BOTTOM\"},\"type\":\"ConnectorPlacement.EquallySpacedRectSide\",\"uuid\":\"40385723-46d7-44c7-bad8-75426342e5d4\"}]},\"type\":\"ConnectorPlacement.EquallySpacedConnector\",\"uuid\":\"3814bf41-4d16-483c-99d1-47665b43720b\"}],\"packageUris\":[\"http://schema.mathworks.com/mf0/Connector/R2020b\"],\"version\":\"1.0\"}"
  joint {1..5} (5 alike) : sm_lib/Joints/Revolute Joint  JointMode=Normal  SenseConstraintForce=off  SenseConstraintForceX=off  SenseConstraintForceY=off  SenseConstraintForceZ=off  SenseConstraintTorque=off  SenseConstraintTorqueX=off  SenseConstraintTorqueY=off  SenseConstraintTorqueZ=off  SenseTotalForce=off  SenseTotalForceX=off  SenseTotalForceY=off  SenseTotalForceZ=off  SenseTotalTorque=off  SenseTotalTorqueX=off  SenseTotalTorqueY=off  SenseTotalTorqueZ=off  CompositeWrenchDir=FollowerOnBase  CompositeWrenchFrame=BaseFrame  EquilibriumPosition=0  EquilibriumPositionUnits=deg  SpringStiffness=internal_stiffness  SpringStiffnessUnits=N*m/deg  DampingCoefficient=0  DampingCoefficientUnits=N*m/(deg/s)  TorqueActuationMode=InputTorque  MotionActuationMode=ComputedMotion  SensePosition=on  SenseVelocity=off  SenseAcceleration=off  SenseTorqueForce=off  SenseLowerLimitTorqueForce=off  SenseUpperLimitTorqueForce=off  LowerLimitSpecify=on  LowerLimitBound=-90  LowerLimitBoundUnits=deg  LowerLimitStiffness=spring_stiffness  LowerLimitStiffnessUnits=N*m/deg  LowerLimitDamping=joint_damp  LowerLimitDampingUnits=N*m/(deg/s)  LowerLimitTransitionRegionWidth=0.1  LowerLimitTransitionRegionWidthUnits=deg  UpperLimitSpecify=on  UpperLimitBound=90  UpperLimitBoundUnits=deg  UpperLimitStiffness=spring_stiffness  UpperLimitStiffnessUnits=N*m/deg  UpperLimitDamping=joint_damp  UpperLimitDampingUnits=N*m/(deg/s)  UpperLimitTransitionRegionWidth=0.1  UpperLimitTransitionRegionWidthUnits=deg  PositionTargetSpecify=off  PositionTargetPriority=High  PositionTargetValue=0  PositionTargetValueUnits=deg  VelocityTargetSpecify=off  VelocityTargetPriority=High  VelocityTargetValue=0  VelocityTargetValueUnits=deg/s
  offset : sm_lib/Frames and Transforms/Rigid Transform  TranslationMethod=Cartesian  TranslationStandardOffset=0  TranslationLengthUnit=m  TranslationStandardAxis=+Z  TranslationCartesianOffset=[0 0 0.06]  TranslationROffset=0  TranslationROffsetUnits=m  TranslationZOffset=0  TranslationZOffsetUnits=m  TranslationThetaOffset=0  TranslationThetaOffsetUnits=deg  RotationMethod=None  RotationAngleUnits=deg  RotationStandardAxis=+Z  RotationAngle=0.0  RotationArbitraryAxis=[0 0 1]  FollAlignAxisA=+X  BaseAlignAxisA=+Y  FollAlignAxisB=+Y  BaseAlignAxisB=+Z  RotationSequenceAxes=FollowerAxes  RotationSequence=XYX  RotationSequenceAngles=[0 0 0]  RotationSequenceAnglesUnits=deg  RotationMatrix=[1 0 0; 0 1 0; 0 0 1]  Quaternion=[1 0 0 0]
  torque control 1 : Subsystem
      settings: PortSchema="{\"entries\":[{\"content\":{\"sides\":[{\"content\":{\"connectorIds\":[\"LConn1\"]},\"type\":\"ConnectorPlacement.EquallySpacedRectSide\",\"uuid\":\"a098fbb4-d319-4217-913e-12f869fe3f7f\"},{\"content\":{\"connectorIds\":[\"RConn1\"],\"side\":\"RIGHT\"},\"type\":\"ConnectorPlacement.EquallySpacedRectSide\",\"uuid\":\"0b47f4a1-f0fa-49d7-9b0e-df1cd63c93cc\"},{\"content\":{\"connectorIds\":[],\"side\":\"TOP\"},\"type\":\"ConnectorPlacement.EquallySpacedRectSide\",\"uuid\":\"12733803-042e-49c1-bd12-ad77a161d0eb\"},{\"content\":{\"connectorIds\":[\"In1\"],\"side\":\"BOTTOM\"},\"type\":\"ConnectorPlacement.EquallySpacedRectSide\",\"uuid\":\"dd4379fb-4796-4e85-9b1d-ab5e12fdce52\"}]},\"type\":\"ConnectorPlacement.EquallySpacedConnector\",\"uuid\":\"2c004d5d-bdbd-4eb1-9300-9454cbe520aa\"}],\"packageUris\":[\"http://schema.mathworks.com/mf0/Connector/R2020b\"],\"version\":\"1.0\"}"
  torque control 2 : Subsystem
      settings: PortSchema="{\"entries\":[{\"content\":{\"sides\":[{\"content\":{\"connectorIds\":[\"LConn1\"]},\"type\":\"ConnectorPlacement.EquallySpacedRectSide\",\"uuid\":\"b601c68f-6f7e-4b60-bd4c-7c9a60dfa343\"},{\"content\":{\"connectorIds\":[\"RConn1\"],\"side\":\"RIGHT\"},\"type\":\"ConnectorPlacement.EquallySpacedRectSide\",\"uuid\":\"26f160aa-f34c-4483-ba01-5c959bffdc56\"},{\"content\":{\"connectorIds\":[],\"side\":\"TOP\"},\"type\":\"ConnectorPlacement.EquallySpacedRectSide\",\"uuid\":\"5bc877b6-64cf-4559-a179-0d622b0df1ec\"},{\"content\":{\"connectorIds\":[\"In1\"],\"side\":\"BOTTOM\"},\"type\":\"ConnectorPlacement.EquallySpacedRectSide\",\"uuid\":\"faa2df67-1e79-4353-a2fd-6cb2d7599dbb\"}]},\"type\":\"ConnectorPlacement.EquallySpacedConnector\",\"uuid\":\"4a9b8871-07f6-45c3-a06e-bcb1a798cb73\"}],\"packageUris\":[\"http://schema.mathworks.com/mf0/Connector/R2020b\"],\"version\":\"1.0\"}"
  torque control 3 : Subsystem
      settings: PortSchema="{\"entries\":[{\"content\":{\"sides\":[{\"content\":{\"connectorIds\":[\"LConn1\"]},\"type\":\"ConnectorPlacement.EquallySpacedRectSide\",\"uuid\":\"a098fbb4-d319-4217-913e-12f869fe3f7f\"},{\"content\":{\"connectorIds\":[\"RConn1\"],\"side\":\"RIGHT\"},\"type\":\"ConnectorPlacement.EquallySpacedRectSide\",\"uuid\":\"0b47f4a1-f0fa-49d7-9b0e-df1cd63c93cc\"},{\"content\":{\"connectorIds\":[],\"side\":\"TOP\"},\"type\":\"ConnectorPlacement.EquallySpacedRectSide\",\"uuid\":\"12733803-042e-49c1-bd12-ad77a161d0eb\"},{\"content\":{\"connectorIds\":[\"In1\"],\"side\":\"BOTTOM\"},\"type\":\"ConnectorPlacement.EquallySpacedRectSide\",\"uuid\":\"25d94116-1506-430a-a4a1-c8171790839f\"}]},\"type\":\"ConnectorPlacement.EquallySpacedConnector\",\"uuid\":\"2c004d5d-bdbd-4eb1-9300-9454cbe520aa\"}],\"packageUris\":[\"http://schema.mathworks.com/mf0/Connector/R2020b\"],\"version\":\"1.0\"}"
  torque control 4 : Subsystem
      settings: PortSchema="{\"entries\":[{\"content\":{\"sides\":[{\"content\":{\"connectorIds\":[\"LConn1\"]},\"type\":\"ConnectorPlacement.EquallySpacedRectSide\",\"uuid\":\"a098fbb4-d319-4217-913e-12f869fe3f7f\"},{\"content\":{\"connectorIds\":[\"RConn1\"],\"side\":\"RIGHT\"},\"type\":\"ConnectorPlacement.EquallySpacedRectSide\",\"uuid\":\"0b47f4a1-f0fa-49d7-9b0e-df1cd63c93cc\"},{\"content\":{\"connectorIds\":[],\"side\":\"TOP\"},\"type\":\"ConnectorPlacement.EquallySpacedRectSide\",\"uuid\":\"12733803-042e-49c1-bd12-ad77a161d0eb\"},{\"content\":{\"connectorIds\":[\"In1\"],\"side\":\"BOTTOM\"},\"type\":\"ConnectorPlacement.EquallySpacedRectSide\",\"uuid\":\"7f35a9b8-c95c-49a8-83ec-cbbfbcbcfe56\"}]},\"type\":\"ConnectorPlacement.EquallySpacedConnector\",\"uuid\":\"2c004d5d-bdbd-4eb1-9300-9454cbe520aa\"}],\"packageUris\":[\"http://schema.mathworks.com/mf0/Connector/R2020b\"],\"version\":\"1.0\"}"
  torque control 5 : Subsystem
      settings: PortSchema="{\"entries\":[{\"content\":{\"sides\":[{\"content\":{\"connectorIds\":[\"LConn1\"]},\"type\":\"ConnectorPlacement.EquallySpacedRectSide\",\"uuid\":\"a098fbb4-d319-4217-913e-12f869fe3f7f\"},{\"content\":{\"connectorIds\":[\"RConn1\"],\"side\":\"RIGHT\"},\"type\":\"ConnectorPlacement.EquallySpacedRectSide\",\"uuid\":\"0b47f4a1-f0fa-49d7-9b0e-df1cd63c93cc\"},{\"content\":{\"connectorIds\":[],\"side\":\"TOP\"},\"type\":\"ConnectorPlacement.EquallySpacedRectSide\",\"uuid\":\"12733803-042e-49c1-bd12-ad77a161d0eb\"},{\"content\":{\"connectorIds\":[\"In1\"],\"side\":\"BOTTOM\"},\"type\":\"ConnectorPlacement.EquallySpacedRectSide\",\"uuid\":\"7f35a9b8-c95c-49a8-83ec-cbbfbcbcfe56\"}]},\"type\":\"ConnectorPlacement.EquallySpacedConnector\",\"uuid\":\"2c004d5d-bdbd-4eb1-9300-9454cbe520aa\"}],\"packageUris\":[\"http://schema.mathworks.com/mf0/Connector/R2020b\"],\"version\":\"1.0\"}"
  xy1 : Outport
  xy2 : Outport  Port=2
  xy3 : Outport  Port=3
  xy4 : Outport  Port=4
  xy5 : Outport  Port=5
  xy6 : Outport  Port=6
  rot1 : Outport  Port=7
  rot2 : Outport  Port=8
  rot3 : Outport  Port=9
  rot4 : Outport  Port=10
  rot5 : Outport  Port=11
  rot6 : Outport  Port=12
  wires:
  Switch1/1 -> Sum2/2
  Sum4/1 -> Scope3/2, torque control 4/1(In1)
  Sine Wave4/1 -> Switch3/1, Divide3/2
  PS-Simulink Converter2/1 -> Scope2/1
  Switch/1 -> Sum1/2
  Sine Wave3/1 -> Switch/1, Divide/2
  Divide3/1 -> Switch3/3
  Clock3/1 -> Switch3/2
  [Bias] -> Sum4/1
  [Bias] -> Sum2/1
  Ramp1/1 -> Divide1/1
  Sum2/1 -> Scope1/2, torque control 2/1(In1)
  Sine Wave1/1 -> Switch1/1, Divide1/2
  PS-Simulink Converter4/1 -> Scope4/1
  Sine Wave5/1 -> Switch4/1, Divide4/2
  Ramp3/1 -> Divide3/1
  Clock1/1 -> Switch1/2
  Divide2/1 -> Switch2/3
  Ramp/1 -> Divide/1
  Divide/1 -> Switch/3
  Clock2/1 -> Switch2/2
  Ramp4/1 -> Divide4/1
  Sum1/1 -> Scope/2, torque control 1/1(In1)
  Sum3/1 -> Scope2/2, torque control 3/1(In1)
  Clock4/1 -> Switch4/2
  Switch3/1 -> Sum4/2
  [Bias] -> Sum1/1
  Divide1/1 -> Switch1/3
  Sum5/1 -> torque control 5/1(In1), Scope4/2
  Ramp2/1 -> Divide2/1
  PS-Simulink Converter/1 -> Scope/1
  PS-Simulink Converter3/1 -> Scope3/1
  Sine Wave2/1 -> Switch2/1, Divide2/2
  Divide4/1 -> Switch4/3
  Clock/1 -> Switch/2
  [Bias] -> Sum3/1
  Switch4/1 -> Sum5/2
  Switch2/1 -> Sum3/2
  PS-Simulink Converter1/1 -> Scope1/1
  [Bias] -> Sum5/1
  body_1/1(rot) -> rot1/1
  body_1/2(xy) -> xy1/1
  body_2/2(xy) -> xy2/1
  body_2/1(rot) -> rot2/1
  body_3/1(rot) -> rot3/1
  body_3/2(xy) -> xy3/1
  body_4/2(xy) -> xy4/1
  body_4/1(rot) -> rot4/1
  body_5/1(rot) -> rot5/1
  body_5/2(xy) -> xy5/1
  body_6/2(xy) -> xy6/1
  body_6/1(rot) -> rot6/1
  Bias/1 -> [Bias]
  connections:
  Rigid Transform4/LConn1 -- joint 1/RConn1
  body_1/RConn1 -- Rigid Transform1/LConn1
  torque control 5/RConn1 -- PS-Simulink Converter4/LConn1 -- joint 5/RConn2
  body_3/LConn1 -- Rigid Transform5/RConn1
  joint 4/LConn1 -- Rigid Transform3/RConn1
  World Frame/RConn1 -- Mechanism Configuration/RConn1 -- Ground/LConn1 -- offset/LConn1 -- Solver Configuration/RConn1
  torque control 4/RConn1 -- PS-Simulink Converter3/LConn1 -- joint 4/RConn2
  joint 2/LConn2 -- torque control 2/LConn1
  Rigid Transform10/LConn1 -- joint 5/RConn1
  torque control 1/RConn1 -- PS-Simulink Converter/LConn1 -- joint 1/RConn2
  torque control 1/LConn1 -- joint 1/LConn2
  joint 4/LConn2 -- torque control 4/LConn1
  6-DOF Joint/LConn1 -- offset/RConn1
  joint 3/RConn2 -- PS-Simulink Converter2/LConn1 -- torque control 3/RConn1
  torque control 2/RConn1 -- PS-Simulink Converter1/LConn1 -- joint 2/RConn2
  Rigid Transform5/LConn1 -- joint 2/RConn1
  joint 3/LConn2 -- torque control 3/LConn1
  body_2/LConn1 -- Rigid Transform4/RConn1
  joint 3/LConn1 -- Rigid Transform7/RConn1
  Rigid Transform6/LConn1 -- joint 4/RConn1
  body_6/LConn1 -- Rigid Transform10/RConn1
  Rigid Transform1/RConn1 -- joint 1/LConn1
  joint 2/LConn1 -- Rigid Transform2/RConn1
  Rigid Transform8/LConn1 -- joint 3/RConn1
  joint 5/LConn1 -- Rigid Transform9/RConn1
  body_1/LConn1 -- 6-DOF Joint/RConn1
  body_2/RConn1 -- Rigid Transform2/LConn1
  joint 5/LConn2 -- torque control 5/LConn1
  body_6/LConn2 -- body_5/LConn2 -- body_4/LConn2 -- body_3/LConn2 -- body_2/LConn2 -- Ground/RConn1 -- body_1/LConn2
  body_4/RConn1 -- Rigid Transform3/LConn1
  body_4/LConn1 -- Rigid Transform8/RConn1
  body_3/RConn1 -- Rigid Transform7/LConn1
  body_5/RConn1 -- Rigid Transform9/LConn1
  body_5/LConn1 -- Rigid Transform6/RConn1
